simulink model "regulateur_pi_discret"  (R2014a)
settings: Solver=ode45  StartTime=0.0  StopTime=1800  RelTol=1e-3
values from neighbouring files (symbols this model uses):
  k = 0.285    [parametres_tp2.m]
  Te = 0.01    [parametres_tp2.m]
  Ti = 100    [parametres_tp2.m]
undefined symbols (not defined in the file or in its folder): DiscIntNeverNeededParam
settings Model: Creator=UTILISATEUR  LastModifiedBy=UTILISATEUR

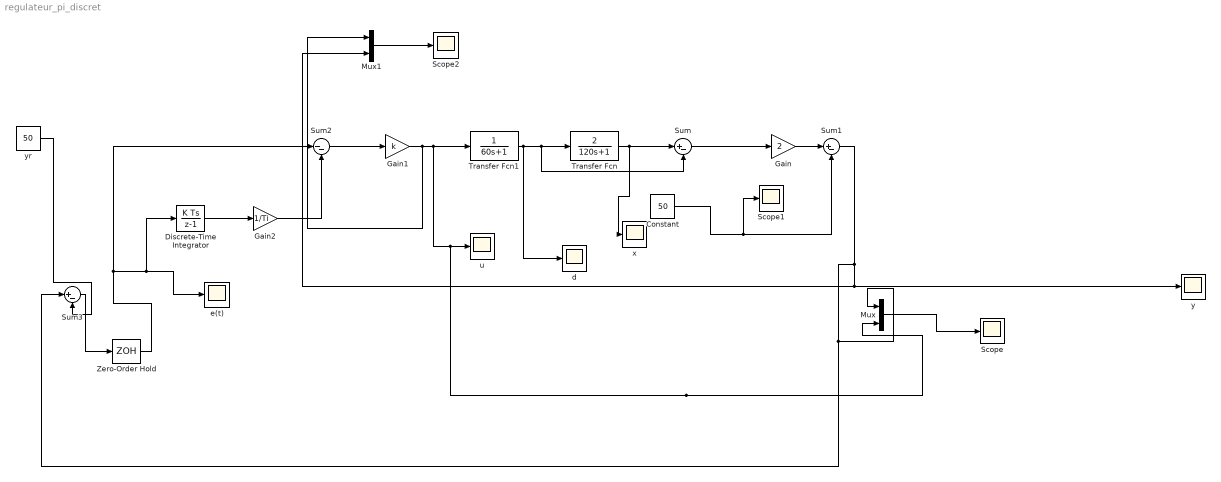
== system regulateur_pi_discret ==
  Constant : Constant  Value=50
  Discrete-Time Integrator : DiscreteIntegrator  SampleTime=Te  ICPrevOutput=DiscIntNeverNeededParam  ICPrevScaledInput=DiscIntNeverNeededParam
  Gain : Gain  Gain=2
  Gain1 : Gain  Gain=k
  Gain2 : Gain  Gain=1/Ti
  Mux : Mux  Inputs=2
  Mux1 : Mux  Inputs=2
  Scope : Scope
      settings: YMin=-500  YMax=500  SaveName=ScopeData2
  Scope1 : Scope
      settings: SaveName=ScopeData3
  Scope2 : Scope
      settings: SaveName=ScopeData4
  Sum : Sum  Inputs=|+-
  Sum1 : Sum  Inputs=|+-
  Sum2 : Sum  Inputs=|--
  Sum3 : Sum  Inputs=|+-
  Transfer Fcn : TransferFcn  Numerator=2  Denominator=[120 1]
  Transfer Fcn1 : TransferFcn  Denominator=[60 1]
  Zero-Order Hold : ZeroOrderHold  SampleTime=Te
  d : Scope
      settings: SaveName=ScopeData5
  e(t) : Scope
      settings: YMin=-120  YMax=120
  u : Scope
      settings: YMin=13.5375  YMax=14.9625  SaveName=ScopeData6
  x : Scope
      settings: SaveName=ScopeData7
  y : Scope
      settings: TimeRange=500  YMin=-100  YMax=200
  "yr " : Constant  Value=50
  wires:
  Transfer Fcn1/1 -> d/1, Sum/2, Transfer Fcn/1
  Sum/1 -> Gain/1
  Transfer Fcn/1 -> x/1, Sum/1
  Constant/1 -> Scope1/1, Sum1/2
  Gain/1 -> Sum1/1
  Sum2/1 -> Gain1/1
  Sum1/1 -> Mux/1, Sum3/1, y/1, Mux1/2
  Gain1/1 -> Mux1/1, Mux/2, u/1, Transfer Fcn1/1
  "yr "/1 -> Sum3/2
  Zero-Order Hold/1 -> Sum2/1, Discrete-Time Integrator/1, e(t)/1
  Mux/1 -> Scope/1
  Discrete-Time Integrator/1 -> Gain2/1
  Gain2/1 -> Sum2/2
  Mux1/1 -> Scope2/1
  Sum3/1 -> Zero-Order Hold/1
